simulink subsystem "PvtSubSys_VSM_UOM"  (R2020b)
settings: Solver=VariableStepAuto  StartTime=0.0  StopTime=10.0  RelTol=1e-3
undefined symbols (not defined in the file or in its folder): P_VSM_ALCSwtReq, P_VSM_PowerTrainConfig
libraries: simulink x9, TrueDurationTime x1
settings Model: Creator=GW00133806  LastModifiedBy=GW00201299

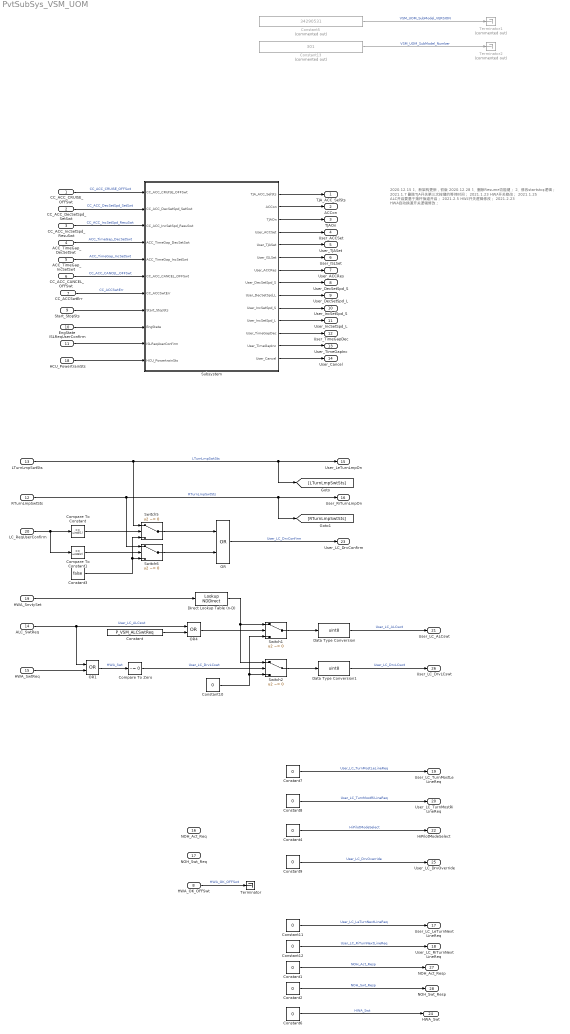
== system PvtSubSys_VSM_UOM ==
  note: 2020.12.15
      | 1、新架构更新，初版
      | 2020.12.28
      | 1、删除Resume功能键；
      | 2、修改startstop逻辑；
      | 2021.1.7
      | 删除TJA开关第三次按键的等待时间；
      | 2021.1.23
      | HWA开关修改；
      | 2021.1.25
      | ALC开启要基于拨杆换道开启；
      | 2021.2.5
      | HWA开关逻辑修改；
      | 2021.2.23
      | HWA自动换道开关逻辑修改；
  CC_ACC_CRUISE_OFFSwt : Inport  OutDataTypeStr=boolean  PortDimensions=1
  CC_ACC_DecSetSpd_SetSwt : Inport  Port=2  OutDataTypeStr=boolean  PortDimensions=1
  CC_ACC_IncSetSpd_ResuSwt : Inport  Port=3  OutDataTypeStr=boolean  PortDimensions=1
  ACC_TimeGap_DecSetSwt : Inport  Port=4  OutDataTypeStr=boolean  PortDimensions=1
  ACC_TimeGap_IncSetSwt : Inport  Port=5  OutDataTypeStr=boolean  PortDimensions=1
  CC_ACC_CANCEL_OFFSwt : Inport  Port=6  OutDataTypeStr=boolean  PortDimensions=1
  CC_ACCSwtErr : Inport  Port=7  OutDataTypeStr=boolean  PortDimensions=1
  HWA_OK_OFFSwt : Inport  Port=8  OutDataTypeStr=boolean  PortDimensions=1
  Start_StopSts : Inport  Port=9  OutDataTypeStr=uint8
  EngState : Inport  Port=10  OutDataTypeStr=uint8
  ISLReqUserConfirm : Inport  Port=11  OutDataTypeStr=boolean
  RTurnLmpSwtSts : Inport  Port=12  OutDataTypeStr=boolean  PortDimensions=1
  LTurnLmpSwtSts : Inport  Port=13  OutDataTypeStr=boolean  PortDimensions=1
  ALC_SwtReq : Inport  Port=14  OutDataTypeStr=boolean
  HWA_SwtReq : Inport  Port=15  OutDataTypeStr=boolean
  NOH_Act_Req : Inport  Port=16
  NOH_Swt_Req : Inport  Port=17
  HCU_PowertrainSts : Inport  Port=18
  HWA_SnvtySet : Inport  Port=19
  LC_ReqUserConfirm : Inport  Port=20  OutDataTypeStr=boolean
  Compare To Constant : simulink/Logic and Bit Operations/Compare To Constant  relop===  const=uint8(1)  OutDataTypeStr=boolean
  Compare To Constant1 : simulink/Logic and Bit Operations/Compare To Constant  relop===  const=uint8(2)  OutDataTypeStr=boolean
  Compare To Zero : simulink/Logic and Bit Operations/Compare To Zero  relop=~=  OutDataTypeStr=uint8
  Constant : Constant  Value=P_VSM_ALCSwtReq
  Constant{1..2,6..8,11..12} (7 alike) : Constant  Value=0  OutDataTypeStr=boolean
  Constant10 : Constant  Value=0  OutDataTypeStr=uint8
  Constant13 : Constant  Commented=on  Value=301  OutDataTypeStr=uint16
  Constant3 : Constant  Value=false
  Constant4 : Constant  Value=0  OutDataTypeStr=uint8
  Constant5 : Constant  Commented=on  Value=34290531  OutDataTypeStr=uint32
  Constant9 : Constant  Value=0  OutDataTypeStr=uint8
  Data Type Conversion : DataTypeConversion  OutDataTypeStr=uint8
  Data Type Conversion1 : DataTypeConversion  OutDataTypeStr=uint8
  Direct Lookup Table (n-D) : LookupNDDirect  NumberOfTableDimensions=1  Table=[2 3 1]  TableDataTypeStr=uint8
  OR : Logic  Operator=OR  AllPortsSameDT=off  OutDataTypeStr=boolean
  OR1 : Logic  Operator=OR  AllPortsSameDT=off  OutDataTypeStr=boolean
  OR4 : Logic  Operator=OR  AllPortsSameDT=off  OutDataTypeStr=boolean
  Subsystem : Subsystem
  Switch{1..2,5..6} (4 alike) : Switch  Criteria=u2 ~= 0
  Terminator : Terminator
  Terminator1 : Terminator  Commented=on
  Terminator2 : Terminator  Commented=on
  TJA_ACC_SelSts : Outport  OutDataTypeStr=uint8
  ACCon : Outport  Port=2  OutDataTypeStr=boolean
  TJAOn : Outport  Port=3  OutDataTypeStr=boolean
  User_ACCSet : Outport  Port=4  OutDataTypeStr=boolean
  User_TJASet : Outport  Port=5  OutDataTypeStr=boolean
  User_ISLSet : Outport  Port=6  OutDataTypeStr=boolean
  User_ACCRes : Outport  Port=7  OutDataTypeStr=boolean
  User_DecSetSpd_S : Outport  Port=8  OutDataTypeStr=boolean
  User_DecSetSpd_L : Outport  Port=9  OutDataTypeStr=boolean
  User_IncSetSpd_S : Outport  Port=10  OutDataTypeStr=boolean
  User_IncSetSpd_L : Outport  Port=11  OutDataTypeStr=boolean
  User_TimeGapDec : Outport  Port=12  OutDataTypeStr=boolean
  User_TimeGapInc : Outport  Port=13  OutDataTypeStr=boolean
  User_Cancel : Outport  Port=14  OutDataTypeStr=boolean
  User_LeTurnLmpOn : Outport  Port=15  OutDataTypeStr=boolean
  User_RiTurnLmpOn : Outport  Port=16  OutDataTypeStr=boolean
  User_LC_LeTurnNextLineReq : Outport  Port=17  OutDataTypeStr=boolean
  User_LC_RiTurnNextLineReq : Outport  Port=18  OutDataTypeStr=boolean
  User_LC_TurnMostLeLineReq : Outport  Port=19  OutDataTypeStr=boolean
  User_LC_TurnMostRiLineReq : Outport  Port=20  OutDataTypeStr=boolean
  User_LC_ALCswt : Outport  Port=21  OutDataTypeStr=uint8
  HiPilotModeSelect : Outport  Port=22  OutDataTypeStr=uint8
  User_LC_DrvConfirm : Outport  Port=23  OutDataTypeStr=boolean
  HWA_Swt : Outport  Port=24  OutDataTypeStr=boolean  PortDimensions=1
  User_LC_DrvOverride : Outport  Port=25  OutDataTypeStr=uint8
  User_LC_DrvLCswt : Outport  Port=26  OutDataTypeStr=uint8
  NOH_Act_Resp : Outport  Port=27
  NOH_Swt_Resp : Outport  Port=28
  wires:
  Constant13/1 -> Terminator2/1  "VSM_UOM_SubModel_Number"
  Constant5/1 -> Terminator1/1  "VSM_UOM_SubModel_VERSION"
  Data Type Conversion1/1 -> User_LC_DrvLCswt/1  "User_LC_DrvLCswt"
  HWA_SwtReq/1 -> OR1/2
  Constant6/1 -> HWA_Swt/1  "HWA_Swt"
  Constant10/1 -> Switch2/3, Switch1/3
  Switch2/1 -> Data Type Conversion1/1
  HCU_PowertrainSts/1 -> Subsystem/11(HCU_PowertrainSts)
  Constant2/1 -> NOH_Swt_Resp/1  "NOH_Swt_Resp"
  Constant1/1 -> NOH_Act_Resp/1  "NOH_Act_Resp"
  Compare To Zero/1 -> Switch2/2  "User_LC_DrvLCswt"
  Constant9/1 -> User_LC_DrvOverride/1  "User_LC_DrvOverride"
  HWA_OK_OFFSwt/1 -> Terminator/1  "HWA_OK_OFFSwt"
  ALC_SwtReq/1 -> OR4/1, OR1/1  "User_LC_ALCswt"
  Constant8/1 -> User_LC_TurnMostRiLineReq/1  "User_LC_TurnMostRiLineReq"
  Constant7/1 -> User_LC_TurnMostLeLineReq/1  "User_LC_TurnMostLeLineReq"
  Switch6/1 -> OR/2
  Constant3/1 -> Switch6/3, Switch5/3
  LTurnLmpSwtSts/1 -> Switch5/1, User_LeTurnLmpOn/1, [LTurnLmpSwtSts]  "LTurnLmpSwtSts"
  Switch5/1 -> OR/1
  Constant/1 -> OR4/2
  Compare To Constant/1 -> Switch5/2
  Compare To Constant1/1 -> Switch6/2
  LC_ReqUserConfirm/1 -> Compare To Constant1/1, Compare To Constant/1
  RTurnLmpSwtSts/1 -> Switch6/1, [RTurnLmpSwtSts], User_RiTurnLmpOn/1  "RTurnLmpSwtSts"
  OR1/1 -> Compare To Zero/1  "HWA_Swt"
  HWA_SnvtySet/1 -> Direct Lookup Table (n-D)/1
  Subsystem/4(User_ACCSet) -> User_ACCSet/1
  CC_ACC_IncSetSpd_ResuSwt/1 -> Subsystem/3(CC_ACC_IncSetSpd_ResuSwt)  "CC_ACC_IncSetSpd_ResuSwt"
  Subsystem/12(User_TimeGapDec) -> User_TimeGapDec/1
  CC_ACC_DecSetSpd_SetSwt/1 -> Subsystem/2(CC_ACC_DecSetSpd_SetSwt)  "CC_ACC_DecSetSpd_SetSwt"
  Subsystem/13(User_TimeGapInc) -> User_TimeGapInc/1
  Subsystem/6(User_ISLSet) -> User_ISLSet/1
  CC_ACC_CRUISE_OFFSwt/1 -> Subsystem/1(CC_ACC_CRUISE_OFFSwt)  "CC_ACC_CRUISE_OFFSwt"
  ACC_TimeGap_IncSetSwt/1 -> Subsystem/5(ACC_TimeGap_IncSetSwt)  "ACC_TimeGap_IncSetSwt"
  ISLReqUserConfirm/1 -> Subsystem/10(ISLReqUserConfirm)
  CC_ACC_CANCEL_OFFSwt/1 -> Subsystem/6(CC_ACC_CANCEL_OFFSwt)  "CC_ACC_CANCEL_OFFSwt"
  ACC_TimeGap_DecSetSwt/1 -> Subsystem/4(ACC_TimeGap_DecSetSwt)  "ACC_TimeGap_DecSetSwt"
  Start_StopSts/1 -> Subsystem/8(Start_StopSts)
  Subsystem/3(TJAOn) -> TJAOn/1
  Subsystem/7(User_ACCRes) -> User_ACCRes/1
  Subsystem/11(User_IncSetSpd_L) -> User_IncSetSpd_L/1
  Subsystem/9(User_DecSetSpd_L) -> User_DecSetSpd_L/1
  Subsystem/5(User_TJASet) -> User_TJASet/1
  EngState/1 -> Subsystem/9(EngState)
  Subsystem/2(ACCon) -> ACCon/1
  CC_ACCSwtErr/1 -> Subsystem/7(CC_ACCSwtErr)  "CC_ACCSwtErr"
  Subsystem/8(User_DecSetSpd_S) -> User_DecSetSpd_S/1
  Subsystem/10(User_IncSetSpd_S) -> User_IncSetSpd_S/1
  Subsystem/14(User_Cancel) -> User_Cancel/1
  Subsystem/1(TJA_ACC_SelSts) -> TJA_ACC_SelSts/1
  Constant4/1 -> HiPilotModeSelect/1  "HiPilotModeSelect"
  OR/1 -> User_LC_DrvConfirm/1  "User_LC_DrvConfirm"
  Data Type Conversion/1 -> User_LC_ALCswt/1  "User_LC_ALCswt"
  Switch1/1 -> Data Type Conversion/1
  OR4/1 -> Switch1/2
  Direct Lookup Table (n-D)/1 -> Switch1/1, Switch2/1
  Constant11/1 -> User_LC_LeTurnNextLineReq/1  "User_LC_LeTurnNextLineReq"
  Constant12/1 -> User_LC_RiTurnNextLineReq/1  "User_LC_RiTurnNextLineReq"

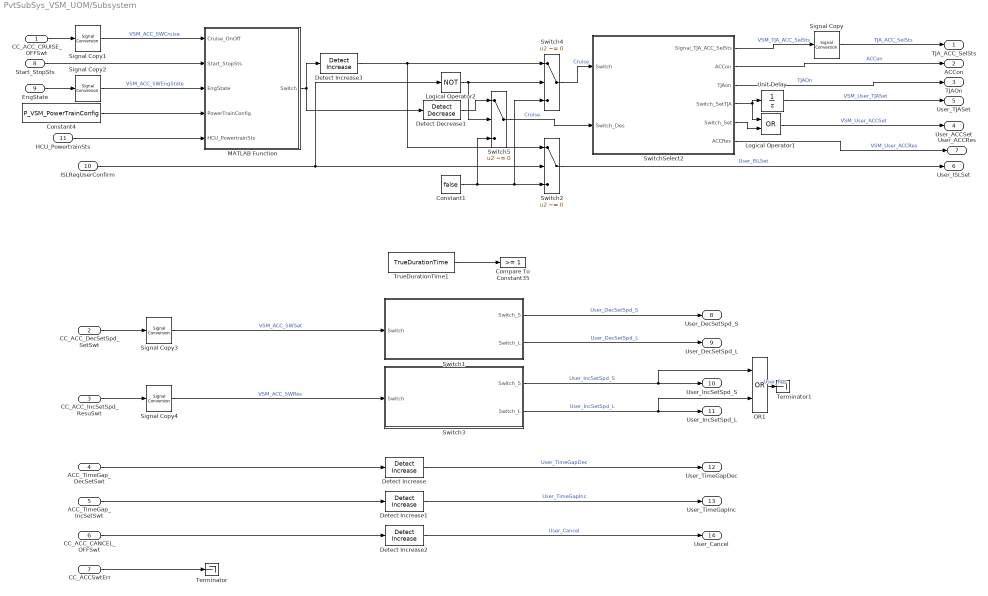
== system PvtSubSys_VSM_UOM/Subsystem ==
  CC_ACC_CRUISE_OFFSwt : Inport  OutDataTypeStr=boolean  PortDimensions=1
  CC_ACC_DecSetSpd_SetSwt : Inport  Port=2  OutDataTypeStr=boolean  PortDimensions=1
  CC_ACC_IncSetSpd_ResuSwt : Inport  Port=3  OutDataTypeStr=boolean  PortDimensions=1
  ACC_TimeGap_DecSetSwt : Inport  Port=4  OutDataTypeStr=boolean  PortDimensions=1
  ACC_TimeGap_IncSetSwt : Inport  Port=5  OutDataTypeStr=boolean  PortDimensions=1
  CC_ACC_CANCEL_OFFSwt : Inport  Port=6  OutDataTypeStr=boolean  PortDimensions=1
  CC_ACCSwtErr : Inport  Port=7  OutDataTypeStr=boolean  PortDimensions=1
  Start_StopSts : Inport  Port=8  OutDataTypeStr=uint8
  EngState : Inport  Port=9  OutDataTypeStr=uint8
  ISLReqUserConfirm : Inport  Port=10  OutDataTypeStr=boolean
  HCU_PowertrainSts : Inport  Port=11
  Compare To Constant35 : simulink/Logic and Bit Operations/Compare To Constant  relop=>=  const=1  OutDataTypeStr=boolean
  Constant1 : Constant  Value=false
  Constant4 : Constant  Value=P_VSM_PowerTrainConfig
  Detect Decrease1 : simulink/Logic and Bit Operations/Detect Decrease  vinit=0.0  OutDataTypeStr=boolean
  Detect Increase{,1..3} (4 alike) : simulink/Logic and Bit Operations/Detect Increase  vinit=0.0  OutDataTypeStr=boolean
  Logical Operator1 : Logic  Operator=OR  AllPortsSameDT=off  OutDataTypeStr=boolean
  Logical Operator2 : Logic  Operator=NOT  Inputs=1  AllPortsSameDT=off  OutDataTypeStr=boolean
  MATLAB Function : MATLAB Function  TreatAsAtomicUnit=on
  OR1 : Logic  Operator=OR  AllPortsSameDT=off  OutDataTypeStr=boolean
  Signal Copy{,1..4} (5 alike) : SignalConversion  OverrideOpt=off
  Switch1 : Stateflow chart  TreatAsAtomicUnit=on
  Switch2 : Switch  Criteria=u2 ~= 0
  Switch3 : Stateflow chart  TreatAsAtomicUnit=on
  Switch4 : Switch  Criteria=u2 ~= 0
  Switch5 : Switch  Criteria=u2 ~= 0
  SwitchSelect2 : Stateflow chart  TreatAsAtomicUnit=on
  Terminator : Terminator
  Terminator1 : Terminator
  TrueDurationTime1 : TrueDurationTime/TrueDurationTime  TCycle=0.02
  Unit Delay : UnitDelay  SampleTime=-1  HasFrameUpgradeWarning=on
  TJA_ACC_SelSts : Outport  OutDataTypeStr=uint8
  ACCon : Outport  Port=2  OutDataTypeStr=boolean
  TJAOn : Outport  Port=3  OutDataTypeStr=boolean
  User_ACCSet : Outport  Port=4  OutDataTypeStr=boolean
  User_TJASet : Outport  Port=5  OutDataTypeStr=boolean
  User_ISLSet : Outport  Port=6  OutDataTypeStr=boolean
  User_ACCRes : Outport  Port=7  OutDataTypeStr=boolean
  User_DecSetSpd_S : Outport  Port=8  OutDataTypeStr=boolean
  User_DecSetSpd_L : Outport  Port=9  OutDataTypeStr=boolean
  User_IncSetSpd_S : Outport  Port=10  OutDataTypeStr=boolean
  User_IncSetSpd_L : Outport  Port=11  OutDataTypeStr=boolean
  User_TimeGapDec : Outport  Port=12  OutDataTypeStr=boolean
  User_TimeGapInc : Outport  Port=13  OutDataTypeStr=boolean
  User_Cancel : Outport  Port=14  OutDataTypeStr=boolean
  wires:
  Switch5/1 -> SwitchSelect2/2(Switch_Des)  "Cruise"
  Detect Decrease1/1 -> Switch5/1
  TrueDurationTime1/1 -> Compare To Constant35/1
  SwitchSelect2/1(Signal_TJA_ACC_SelSts) -> Signal Copy/1  "VSM_TJA_ACC_SelSts"
  Switch1/1(Switch_S) -> User_DecSetSpd_S/1  "User_DecSetSpd_S"
  SwitchSelect2/6(ACCRes) -> User_ACCRes/1  "VSM_User_ACCRes"
  Logical Operator1/1 -> User_ACCSet/1  "VSM_User_ACCSet"
  Detect Increase2/1 -> User_Cancel/1  "User_Cancel"
  ACC_TimeGap_IncSetSwt/1 -> Detect Increase1/1
  CC_ACCSwtErr/1 -> Terminator/1
  SwitchSelect2/3(TJAon) -> TJAOn/1  "TJAOn"
  Signal Copy1/1 -> MATLAB Function/1(Cruise_OnOff)  "VSM_ACC_SWCruise"
  Switch3/2(Switch_L) -> OR1/2, User_IncSetSpd_L/1  "User_IncSetSpd_L"
  Switch1/2(Switch_L) -> User_DecSetSpd_L/1  "User_DecSetSpd_L"
  CC_ACC_CANCEL_OFFSwt/1 -> Detect Increase2/1
  SwitchSelect2/2(ACCon) -> ACCon/1  "ACCon"
  ISLReqUserConfirm/1 -> Switch2/2, Logical Operator2/1
  Start_StopSts/1 -> MATLAB Function/2(Start_StopSts)
  Switch3/1(Switch_S) -> OR1/1, User_IncSetSpd_S/1  "User_IncSetSpd_S"
  Switch4/1 -> SwitchSelect2/1(Switch)  "Cruise"
  MATLAB Function/1(Switch) -> Detect Decrease1/1, Detect Increase3/1
  Switch2/1 -> User_ISLSet/1  "User_ISLSet"
  Detect Increase1/1 -> User_TimeGapInc/1  "User_TimeGapInc"
  CC_ACC_IncSetSpd_ResuSwt/1 -> Signal Copy4/1
  Signal Copy/1 -> TJA_ACC_SelSts/1  "TJA_ACC_SelSts"
  SwitchSelect2/5(Switch_Set) -> Logical Operator1/2
  Detect Increase/1 -> User_TimeGapDec/1  "User_TimeGapDec"
  ACC_TimeGap_DecSetSwt/1 -> Detect Increase/1
  SwitchSelect2/4(Switch_SetTJA) -> Unit Delay/1, Logical Operator1/1
  Logical Operator2/1 -> Switch5/2, Switch4/2
  Constant1/1 -> Switch4/3, Switch2/3, Switch5/3
  Signal Copy3/1 -> Switch1/1(Switch)  "VSM_ACC_SWSet"
  Detect Increase3/1 -> Switch2/1, Switch4/1
  Signal Copy2/1 -> MATLAB Function/3(EngState)  "VSM_ACC_SWEngState"
  Unit Delay/1 -> User_TJASet/1  "VSM_User_TJASet"
  CC_ACC_CRUISE_OFFSwt/1 -> Signal Copy1/1
  EngState/1 -> Signal Copy2/1
  CC_ACC_DecSetSpd_SetSwt/1 -> Signal Copy3/1
  Signal Copy4/1 -> Switch3/1(Switch)  "VSM_ACC_SWRes"
  OR1/1 -> Terminator1/1  "User_Res"
  Constant4/1 -> MATLAB Function/4(PowerTrainConfig)
  HCU_PowertrainSts/1 -> MATLAB Function/5(HCU_PowertrainSts)

== matlab function PvtSubSys_VSM_UOM/Subsystem/MATLAB Function ==
  data: Cruise_OnOff input; Switch output boolean; Start_StopSts input; EngState input; PowerTrainConfig input; HCU_PowertrainSts input
function Switch = fcn(Cruise_OnOff,Start_StopSts,EngState, PowerTrainConfig, HCU_PowertrainSts)
%#codegen
if PowerTrainConfig == 0
    if ((Start_StopSts==0 || Start_StopSts==1 || Start_StopSts==7) && EngState==0)
        Switch = false;
    else
        Switch = Cruise_OnOff;
    end
else
    if HCU_PowertrainSts == 5
       Switch = Cruise_OnOff;
    else
       Switch = false;
    end
end

== stateflow chart PvtSubSys_VSM_UOM/Subsystem/Switch1 ==
  state falling
    en:
    Switch_L=false;
    du:
    Switch_S=false;
  state rising
    en:
    Cnt=0;
    Switch_S=false;
    Switch_L=false;
    du:
    Cnt=min(Cnt+1,3001);
    Switch_L=(Cnt%%50==0);
  (default) -> falling
  (junction 414) -> falling
  falling -> rising : [Switch==1]
  (junction 413) -> falling [order 2] : {Switch_S=true;}
  (junction 413) -> (junction 414) [order 1] : [Cnt>49]
  rising -> (junction 413) : [Switch==0]
  data: Switch_S output boolean =false; Switch_L output boolean =false; Switch input boolean; Cnt local uint16

== stateflow chart PvtSubSys_VSM_UOM/Subsystem/Switch3 ==
  state falling
    en:
    Switch_L=false;
    du:
    Switch_S=false;
  state rising
    en:
    Cnt=0;
    Switch_S=false;
    Switch_L=false;
    du:
    Cnt=min(Cnt+1,3001);
    Switch_L=(Cnt%%50==0);
  (default) -> falling
  (junction 414) -> falling
  falling -> rising : [Switch==1]
  (junction 413) -> falling [order 2] : {Switch_S=true;}
  (junction 413) -> (junction 414) [order 1] : [Cnt>49]
  rising -> (junction 413) : [Switch==0]
  data: Switch_S output boolean =false; Switch_L output boolean =false; Switch input boolean; Cnt local uint16

== stateflow chart PvtSubSys_VSM_UOM/Subsystem/SwitchSelect2 ==
  note: 信号：TJA_ACC_SelSts
      | 0x0:off （Off selected）
      | 0x1:ACC selected
      | 0x2:TJA/ICA selected
      | 0x3:Off selected（Off）
      | 0x4:ACC on
      | 0x5:TJA/ICA on
      | 0x6-0x7:Reserved
  state notpress
    Cntlive=0;
    Switch_Set=false;
    Switch_SetTJA=false;
    ACCRes = false;
  state Click
    Cntlive=min(Cntlive+1,200);
    ex:
    Cntlive=0;
  state Res
    ACCRes=true;
    Cntlive=min(Cntlive+1,200);
    ex:
    Cntlive=0;
  state SetACC
    Switch_Set=true;
    Cntlive=min(Cntlive+1,200);
  state DoubleClickWait
    Cntlive=min(Cntlive+1,200);
    ex:
    Cntlive=0;
  state DoubleClick
  state SetTJA
    Switch_SetTJA=true;
    Cntlive=min(Cntlive+1,200);
  state Triple_ClickWait [commented out]
    Cntlive=min(Cntlive+1,200);
    ex:
    Cntlive=0;
  (default) -> notpress : {ACCon=true;
      | TJAon=true;
      | Signal_TJA_ACC_SelSts=2;}
  notpress -> Click : [Switch]
  Res -> notpress : [Cntlive>1]
  SetACC -> notpress : [Cntlive>1]
  SetTJA -> notpress : [Cntlive>1]
  Click -> Res [order 2] : [Cntlive>=50&&[Switch_Des]]
  Click -> DoubleClickWait [order 1] : [Switch_Des&&Cntlive<50]
  DoubleClickWait -> SetACC [order 1] : [Cntlive>25]
  DoubleClickWait -> DoubleClick [order 2] : [Switch]
  DoubleClick -> SetTJA : [~Switch]
  Triple_ClickWait -> ? [commented out] : [Cntlive>25]
  data: Cntlive local size=1; Signal_TJA_ACC_SelSts output uint8 size=1; Switch input boolean size=1; ACCon output boolean; TJAon output boolean; Switch_SetTJA output boolean; Switch_Set output boolean; Switch_Des input; ACCRes output
